simulink library "siltestlib"  (Simulink 5.2)
settings Model: LastModifiedBy=srd  ExtModeMexFile=rti_comm  ExtModeArmWhenConnect=off  ProdHWDeviceType=Microprocessor  RTWMakeCommand=make_rti  RTWRetainRTWFile=on

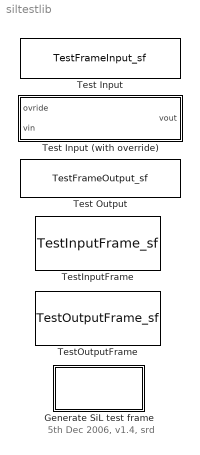
== system siltestlib ==
  note: 5th Dec 2006, v1.4, srd
  Generate SiL test frame : Subsystem  Description=Generate SiL\ntest frame  TreatAsAtomicUnit=on
      settings: OpenFcn=|
      | if exist('gen_sil_test_frame','file'), gen_sil_test_frame(gcs); else,
      | fprintf('Error: gen_sil_test_frame is not on the matlab path.\n'); end
      mask Type: Generate SiL test frame button.
      mask Description: Calls the function gen_sil_test_frame.
      mask Help: Calls the function gen_sil_test_frame.
      mask Display: fprintf('Generate SiL\ntest frame');
  Test Input : S-Function  FunctionName=TestFrameInput_sf  Parameters=varname,sampletime  mask(Test Input){varname=<UNDEFINED>, sampletime=-1}
      mask prompts: varname "Name:"; sampletime "Sample Time:"
      mask help: Outputs the value of a Test Input variable from an Excel spreadsheet when used with the runsiltest script. Otherwise outputs 0.
      mask Display: fprintf('Test Input:\n%s',varname);
  Test Input (with override) : Subsystem  mask(Test Input (with override)){varname=<UNDEFINED>, sampletime=-1}
      mask prompts: varname "Name:"; sampletime "Sample Time:"
      mask help: Outputs the input value if ovride >= 0.5 otherwise outputs the value from the SiLTest frame in the Matlab workspace. If not present then outputs 0.
      mask Help: Outputs the input value if ovride >= 0.5 otherwise outputs the value from the SiLTest frame in the Matlab workspace. If not present then outputs 0.
      mask Display:
      | fprintf('Test Input\n(with override):\n%s',varname);
      | port_label('input', 1, 'ovride')
      | port_label('input', 2, 'vin')
      | port_label('output', 1, 'vout')
  Test Output : S-Function  FunctionName=TestFrameOutput_sf  Parameters=varname,sampletime  mask(Test Output){varname=<UNDEFINED>, sampletime=-1}
      mask prompts: varname "Name:"; sampletime "Sample Time:"
      mask help: Samples the value of a Test Output variable from an Excel spreadsheet when used with the runsiltest script. Otherwise does nothing.
      mask Display: fprintf('Test Output:\n%s',varname);
  TestInputFrame : S-Function  FunctionName=TestInputFrame_sf
      mask Type: TestInputFrame
      mask Description:
      | Set the value of the obd array in Matlab from obdset input variables.
      | Update Matlab calibration from cal inputs.
      mask Help:
      | Set the value of the obd array in Matlab from obdset input variables.
      | Update Matlab calibration from cal inputs.
      mask Display: fprintf('TestInputFrame');
  TestOutputFrame : S-Function  FunctionName=TestOutputFrame_sf
      mask Type: TestOutputFrame
      mask Description: Sets the value of obdget output variables from the obd array in Matlab.
      mask Help: Sets the value of obdget output variables from the obd array in Matlab.
      mask Display: fprintf('TestOutputFrame');

== system siltestlib/Generate SiL test frame ==

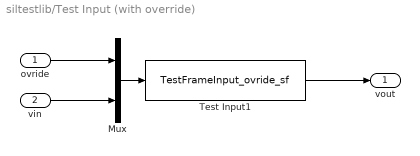
== system siltestlib/Test Input (with override) ==
  ovride : Inport
  vin : Inport  Port=2
  Mux : Mux  Inputs=2
  Test Input1 : S-Function  FunctionName=TestFrameInput_ovride_sf  Parameters=varname,sampletime
  vout : Outport
  wires:
  vin/1 -> Mux/2
  ovride/1 -> Mux/1
  Mux/1 -> Test Input1/1
  Test Input1/1 -> vout/1
